simulink model "modelado_testing"  (R2021a)
settings: Solver=VariableStepAuto  StartTime=0.0  StopTime=10.0  RelTol=1e-3
settings Model: Creator=marcu  LastModifiedBy=marcu

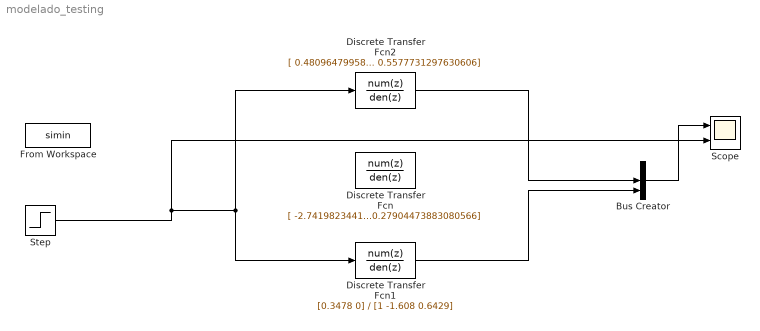
== system modelado_testing ==
  Bus Creator : BusCreator  Inputs=3
  Discrete Transfer Fcn : DiscreteTransferFcn  Numerator=[ -2.7419823441194717 3.788184230895976 ]  Denominator=[1 -1.1737430252296377 0.27904473883080566]
  Discrete Transfer Fcn1 : DiscreteTransferFcn  Numerator=[0.3478 0]  Denominator=[1 -1.608 0.6429]
  Discrete Transfer Fcn2 : DiscreteTransferFcn  Numerator=[ 0.48096479958008587 0]  Denominator=[1 -1.5093644009548426 0.5577731297630606]
  From Workspace : FromWorkspace  VariableName=simin
  Scope : Scope  NumInputPorts=2
  Step : Step  After=3  SampleTime=0.01
  wires:
  Step/1 -> Scope/2, Discrete Transfer Fcn2/1, Discrete Transfer Fcn1/1
  Bus Creator/1 -> Scope/1
  Discrete Transfer Fcn1/1 -> Bus Creator/3
  Discrete Transfer Fcn2/1 -> Bus Creator/2
